simulink model "c00017M_harness"  (R2018a)
settings: Solver=FixedStepAuto  StartTime=0.0  StopTime=300  FixedStep=0.1  RelTol=1e-3
undefined symbols (not defined in the file): A1, hmax, R1, R2, sigbuilder_block
(part 1 of 6)
settings Model: Creator=aarrieta  LastModifiedBy=umarkiegi

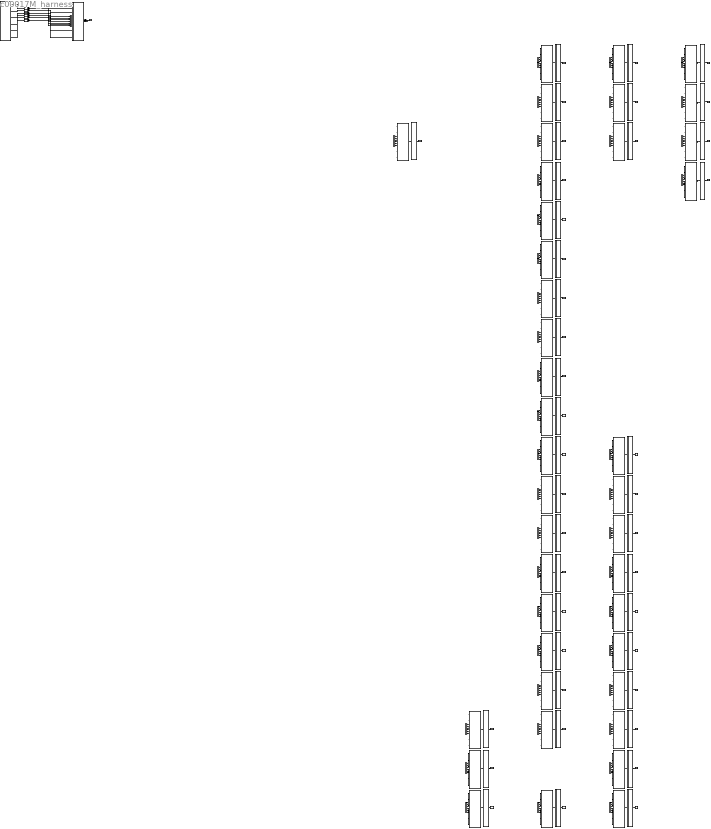
== system c00017M_harness ==
  CPSUT : Subsystem
  Eval117 : Subsystem
  Eval118 : Subsystem
  Eval119 : Subsystem
  Eval120 : Subsystem
  Eval121 : Subsystem
  Eval122 : Subsystem
  Eval123 : Subsystem
  Eval124 : Subsystem
  Eval125 : Subsystem
  Eval126 : Subsystem
  Eval127 : Subsystem
  Eval128 : Subsystem
  Eval129 : Subsystem
  Eval130 : Subsystem
  Eval131 : Subsystem
  Eval132 : Subsystem
  Eval133 : Subsystem
  Eval134 : Subsystem
  Eval135 : Subsystem
  Eval136 : Subsystem
  Eval137 : Subsystem
  Eval139 : Subsystem
  Eval140 : Subsystem
  Eval141 : Subsystem
  Eval142 : Subsystem
  Eval150 : Subsystem
  Eval151 : Subsystem
  Eval152 : Subsystem
  Eval153 : Subsystem
  Eval154 : Subsystem
  Eval155 : Subsystem
  Eval156 : Subsystem
  Eval157 : Subsystem
  Eval158 : Subsystem
  Eval159 : Subsystem
  Eval160 : Subsystem
  Eval161 : Subsystem
  Eval162 : Subsystem
  Eval163 : Subsystem
  Eval82 : Subsystem
  Inputs : Subsystem  Tag=STV Subsys  LoadFcn=sigbuilder_block('load');  StartFcn=sigbuilder_block('start');  StopFcn=sigbuilder_block('stop');  ClipboardFcn=sigbuilder_block('clipboard');  mask(Sigbuilder block){tuvar=[0:10]}
      mask init:
      | if ~strcmp(get_param(bdroot(gcb),'SimulationStatus'),'stopped'),tuvar = sigbuilder_block('maskInit'); end
      settings: CopyFcn=sigbuilder_block('copy');  DeleteFcn=sigbuilder_block('delete');  ModelCloseFcn=sigbuilder_block('modelClose');  PreSaveFcn=sigbuilder_block('preSave');  PauseFcn=sigbuilder_block('pause');  ContinueFcn=sigbuilder_block('continue');  NameChangeFcn=sigbuilder_block('namechange');  OpenFcn=sigbuilder_block('open',[276.75 163.5 675.75 486.75 ]);  CloseFcn=sigbuilder_block('close');
      mask Display: plot(0, 0, 100, 100,[2, 2, 32, 32, 2], [68, 8, 8, 68, 68],[32, 2], [38, 38], [32, 19, 2],[53, 60, 44], [32, 17, 17, 2],[16, 16, 31, 31]);txt = getActiveGroup(gcbh);text(2, 100, txt,'verticalAlignment', 'top');
  M083 : Subsystem
  M118 : Subsystem
  M119 : Subsystem
  M120 : Subsystem
  M121 : Subsystem
  M122 : Subsystem
  M123 : Subsystem
  M124 : Subsystem
  M125 : Subsystem
  M126 : Subsystem
  M127 : Subsystem
  M128 : Subsystem
  M129 : Subsystem
  M130 : Subsystem
  M131 : Subsystem
  M132 : Subsystem
  M133 : Subsystem
  M134 : Subsystem
  M135 : Subsystem
  M136 : Subsystem
  M137 : Subsystem
  M138 : Subsystem
  M140 : Subsystem
  M141 : Subsystem
  M142 : Subsystem
  M143 : Subsystem
  M151 : Subsystem
  M152 : Subsystem
  M153 : Subsystem
  M154 : Subsystem
  M155 : Subsystem
  M156 : Subsystem
  M157 : Subsystem
  M158 : Subsystem
  M159 : Subsystem
  M160 : Subsystem
  M161 : Subsystem
  M162 : Subsystem
  M163 : Subsystem
  M164 : Subsystem
  To Workspace117 : ToWorkspace  VariableName=mutant118  SampleTime=-1
  To Workspace118 : ToWorkspace  VariableName=mutant119  SampleTime=-1
  To Workspace119 : ToWorkspace  VariableName=mutant120  SampleTime=-1
  To Workspace120 : ToWorkspace  VariableName=mutant121  SampleTime=-1
  To Workspace121 : ToWorkspace  VariableName=mutant122  SampleTime=-1
  To Workspace122 : ToWorkspace  VariableName=mutant123  SampleTime=-1
  To Workspace123 : ToWorkspace  VariableName=mutant124  SampleTime=-1
  To Workspace124 : ToWorkspace  VariableName=mutant125  SampleTime=-1
  To Workspace125 : ToWorkspace  VariableName=mutant126  SampleTime=-1
  To Workspace126 : ToWorkspace  VariableName=mutant127  SampleTime=-1
  To Workspace127 : ToWorkspace  VariableName=mutant128  SampleTime=-1
  To Workspace128 : ToWorkspace  VariableName=mutant129  SampleTime=-1
  To Workspace129 : ToWorkspace  VariableName=mutant130  SampleTime=-1
  To Workspace130 : ToWorkspace  VariableName=mutant131  SampleTime=-1
  To Workspace131 : ToWorkspace  VariableName=mutant132  SampleTime=-1
  To Workspace132 : ToWorkspace  VariableName=mutant133  SampleTime=-1
  To Workspace133 : ToWorkspace  VariableName=mutant134  SampleTime=-1
  To Workspace134 : ToWorkspace  VariableName=mutant135  SampleTime=-1
  To Workspace135 : ToWorkspace  VariableName=mutant136  SampleTime=-1
  To Workspace136 : ToWorkspace  VariableName=mutant137  SampleTime=-1
  To Workspace137 : ToWorkspace  VariableName=mutant138  SampleTime=-1
  To Workspace139 : ToWorkspace  VariableName=mutant140  SampleTime=-1
  To Workspace140 : ToWorkspace  VariableName=mutant141  SampleTime=-1
  To Workspace141 : ToWorkspace  VariableName=mutant142  SampleTime=-1
  To Workspace142 : ToWorkspace  VariableName=mutant143  SampleTime=-1
  To Workspace150 : ToWorkspace  VariableName=mutant151  SampleTime=-1
  To Workspace151 : ToWorkspace  VariableName=mutant152  SampleTime=-1
  To Workspace152 : ToWorkspace  VariableName=mutant153  SampleTime=-1
  To Workspace153 : ToWorkspace  VariableName=mutant154  SampleTime=-1
  To Workspace154 : ToWorkspace  VariableName=mutant155  SampleTime=-1
  To Workspace155 : ToWorkspace  VariableName=mutant156  SampleTime=-1
  To Workspace156 : ToWorkspace  VariableName=mutant157  SampleTime=-1
  To Workspace157 : ToWorkspace  VariableName=mutant158  SampleTime=-1
  To Workspace158 : ToWorkspace  VariableName=mutant159  SampleTime=-1
  To Workspace159 : ToWorkspace  VariableName=mutant160  SampleTime=-1
  To Workspace160 : ToWorkspace  VariableName=mutant161  SampleTime=-1
  To Workspace161 : ToWorkspace  VariableName=mutant162  SampleTime=-1
  To Workspace162 : ToWorkspace  VariableName=mutant163  SampleTime=-1
  To Workspace163 : ToWorkspace  VariableName=mutant164  SampleTime=-1
  To Workspace82 : ToWorkspace  VariableName=mutant083  SampleTime=-1
  dtc_CT2 : DataTypeConversion
  dtc_E2 : DataTypeConversion
  dtc_EB2 : DataTypeConversion
  dtc_F2 : DataTypeConversion
  dtc_MR2 : DataTypeConversion
  dtc_T2 : DataTypeConversion
  LL2 : Outport
  tag scope: out2=global
  wires:
  CPSUT/1(LL2) -> [out2], LL2/1
  [in7] -> M083/1(CT2)
  [in8] -> M083/2(F2)
  [in9] -> M083/3(E2)
  [in10] -> M083/4(MR2)
  [in11] -> M083/5(T2)
  [in12] -> M083/6(EB2)
  M083/1(LL2) -> Eval82/1(In2)
  Eval82/1(Out1) -> To Workspace82/1
  [in7] -> M118/1(CT2)
  [in8] -> M118/2(F2)
  [in9] -> M118/3(E2)
  [in10] -> M118/4(MR2)
  [in11] -> M118/5(T2)
  [in12] -> M118/6(EB2)
  M118/1(LL2) -> Eval117/1(In2)
  Eval117/1(Out1) -> To Workspace117/1
  [in7] -> M119/1(CT2)
  [in8] -> M119/2(F2)
  [in9] -> M119/3(E2)
  [in10] -> M119/4(MR2)
  [in11] -> M119/5(T2)
  [in12] -> M119/6(EB2)
  M119/1(LL2) -> Eval118/1(In2)
  Eval118/1(Out1) -> To Workspace118/1
  [in7] -> M120/1(CT2)
  [in8] -> M120/2(F2)
  [in9] -> M120/3(E2)
  [in10] -> M120/4(MR2)
  [in11] -> M120/5(T2)
  [in12] -> M120/6(EB2)
  M120/1(LL2) -> Eval119/1(In2)
  Eval119/1(Out1) -> To Workspace119/1
  [in7] -> M121/1(CT2)
  [in8] -> M121/2(F2)
  [in9] -> M121/3(E2)
  [in10] -> M121/4(MR2)
  [in11] -> M121/5(T2)
  [in12] -> M121/6(EB2)
  M121/1(LL2) -> Eval120/1(In2)
  Eval120/1(Out1) -> To Workspace120/1
  [in7] -> M122/1(CT2)
  [in8] -> M122/2(F2)
  [in9] -> M122/3(E2)
  [in10] -> M122/4(MR2)
  [in11] -> M122/5(T2)
  [in12] -> M122/6(EB2)
  M122/1(LL2) -> Eval121/1(In2)
  Eval121/1(Out1) -> To Workspace121/1
  [in7] -> M123/1(CT2)
  [in8] -> M123/2(F2)
  [in9] -> M123/3(E2)
  [in10] -> M123/4(MR2)
  [in11] -> M123/5(T2)
  [in12] -> M123/6(EB2)
  M123/1(LL2) -> Eval122/1(In2)
  Eval122/1(Out1) -> To Workspace122/1
  [in7] -> M124/1(CT2)
  [in8] -> M124/2(F2)
  [in9] -> M124/3(E2)
  [in10] -> M124/4(MR2)
  [in11] -> M124/5(T2)
  [in12] -> M124/6(EB2)
  M124/1(LL2) -> Eval123/1(In2)
  Eval123/1(Out1) -> To Workspace123/1
  [in7] -> M125/1(CT2)
  [in8] -> M125/2(F2)
  [in9] -> M125/3(E2)
  [in10] -> M125/4(MR2)
  [in11] -> M125/5(T2)
  [in12] -> M125/6(EB2)
  M125/1(LL2) -> Eval124/1(In2)
  Eval124/1(Out1) -> To Workspace124/1
  [in7] -> M126/1(CT2)
  [in8] -> M126/2(F2)
  [in9] -> M126/3(E2)
  [in10] -> M126/4(MR2)
  [in11] -> M126/5(T2)
  [in12] -> M126/6(EB2)
  M126/1(LL2) -> Eval125/1(In2)
  Eval125/1(Out1) -> To Workspace125/1
  [in7] -> M127/1(CT2)
  [in8] -> M127/2(F2)
  [in9] -> M127/3(E2)
  [in10] -> M127/4(MR2)
  [in11] -> M127/5(T2)
  [in12] -> M127/6(EB2)
  M127/1(LL2) -> Eval126/1(In2)
  Eval126/1(Out1) -> To Workspace126/1
  [in7] -> M128/1(CT2)
  [in8] -> M128/2(F2)
  [in9] -> M128/3(E2)
  [in10] -> M128/4(MR2)
  [in11] -> M128/5(T2)
  [in12] -> M128/6(EB2)
  M128/1(LL2) -> Eval127/1(In2)
  Eval127/1(Out1) -> To Workspace127/1
  [in7] -> M129/1(CT2)
  [in8] -> M129/2(F2)
  [in9] -> M129/3(E2)
  [in10] -> M129/4(MR2)
  [in11] -> M129/5(T2)
  [in12] -> M129/6(EB2)
  M129/1(LL2) -> Eval128/1(In2)
  Eval128/1(Out1) -> To Workspace128/1
  [in7] -> M130/1(CT2)
  [in8] -> M130/2(F2)
  [in9] -> M130/3(E2)
  [in10] -> M130/4(MR2)
  [in11] -> M130/5(T2)
  [in12] -> M130/6(EB2)
  M130/1(LL2) -> Eval129/1(In2)
  Eval129/1(Out1) -> To Workspace129/1
  [in7] -> M131/1(CT2)
  [in8] -> M131/2(F2)
  [in9] -> M131/3(E2)
  [in10] -> M131/4(MR2)
  [in11] -> M131/5(T2)
  [in12] -> M131/6(EB2)
  M131/1(LL2) -> Eval130/1(In2)
  Eval130/1(Out1) -> To Workspace130/1
  [in7] -> M132/1(CT2)
  [in8] -> M132/2(F2)
  [in9] -> M132/3(E2)
  [in10] -> M132/4(MR2)
  [in11] -> M132/5(T2)
  [in12] -> M132/6(EB2)
  M132/1(LL2) -> Eval131/1(In2)
  Eval131/1(Out1) -> To Workspace131/1
  [in7] -> M133/1(CT2)
  [in8] -> M133/2(F2)
  [in9] -> M133/3(E2)
  [in10] -> M133/4(MR2)
  [in11] -> M133/5(T2)
  [in12] -> M133/6(EB2)
  M133/1(LL2) -> Eval132/1(In2)
  Eval132/1(Out1) -> To Workspace132/1
  [in7] -> M134/1(CT2)
  [in8] -> M134/2(F2)
  [in9] -> M134/3(E2)
  [in10] -> M134/4(MR2)
  [in11] -> M134/5(T2)
  [in12] -> M134/6(EB2)
  M134/1(LL2) -> Eval133/1(In2)
  Eval133/1(Out1) -> To Workspace133/1
  [in7] -> M135/1(CT2)
  [in8] -> M135/2(F2)
  [in9] -> M135/3(E2)
  [in10] -> M135/4(MR2)
  [in11] -> M135/5(T2)
  [in12] -> M135/6(EB2)
  M135/1(LL2) -> Eval134/1(In2)
  Eval134/1(Out1) -> To Workspace134/1
  [in7] -> M136/1(CT2)
  [in8] -> M136/2(F2)
  [in9] -> M136/3(E2)
  [in10] -> M136/4(MR2)
  [in11] -> M136/5(T2)
  [in12] -> M136/6(EB2)
  M136/1(LL2) -> Eval135/1(In2)
  Eval135/1(Out1) -> To Workspace135/1
  [in7] -> M137/1(CT2)
  [in8] -> M137/2(F2)
  [in9] -> M137/3(E2)
  [in10] -> M137/4(MR2)
  [in11] -> M137/5(T2)
  [in12] -> M137/6(EB2)
  M137/1(LL2) -> Eval136/1(In2)
  Eval136/1(Out1) -> To Workspace136/1
  [in7] -> M138/1(CT2)
  [in8] -> M138/2(F2)
  [in9] -> M138/3(E2)
  [in10] -> M138/4(MR2)
  [in11] -> M138/5(T2)
  [in12] -> M138/6(EB2)
  M138/1(LL2) -> Eval137/1(In2)
  Eval137/1(Out1) -> To Workspace137/1
  [in7] -> M140/1(CT2)
  [in8] -> M140/2(F2)
  [in9] -> M140/3(E2)
  [in10] -> M140/4(MR2)
  [in11] -> M140/5(T2)
  [in12] -> M140/6(EB2)
  M140/1(LL2) -> Eval139/1(In2)
  Eval139/1(Out1) -> To Workspace139/1
  [in7] -> M141/1(CT2)
  [in8] -> M141/2(F2)
  [in9] -> M141/3(E2)
  [in10] -> M141/4(MR2)
  [in11] -> M141/5(T2)
  [in12] -> M141/6(EB2)
  M141/1(LL2) -> Eval140/1(In2)
  Eval140/1(Out1) -> To Workspace140/1
  [in7] -> M142/1(CT2)
  [in8] -> M142/2(F2)
  [in9] -> M142/3(E2)
  [in10] -> M142/4(MR2)
  [in11] -> M142/5(T2)
  [in12] -> M142/6(EB2)
  M142/1(LL2) -> Eval141/1(In2)
  Eval141/1(Out1) -> To Workspace141/1
  [in7] -> M143/1(CT2)
  [in8] -> M143/2(F2)
  [in9] -> M143/3(E2)
  [in10] -> M143/4(MR2)
  [in11] -> M143/5(T2)
  [in12] -> M143/6(EB2)
  M143/1(LL2) -> Eval142/1(In2)
  Eval142/1(Out1) -> To Workspace142/1
  [in7] -> M151/1(CT2)
  [in8] -> M151/2(F2)
  [in9] -> M151/3(E2)
  [in10] -> M151/4(MR2)
  [in11] -> M151/5(T2)
  [in12] -> M151/6(EB2)
  M151/1(LL2) -> Eval150/1(In2)
  Eval150/1(Out1) -> To Workspace150/1
  [in7] -> M152/1(CT2)
  [in8] -> M152/2(F2)
  [in9] -> M152/3(E2)
  [in10] -> M152/4(MR2)
  [in11] -> M152/5(T2)
  [in12] -> M152/6(EB2)
  M152/1(LL2) -> Eval151/1(In2)
  Eval151/1(Out1) -> To Workspace151/1
  [in7] -> M153/1(CT2)
  [in8] -> M153/2(F2)
  [in9] -> M153/3(E2)
  [in10] -> M153/4(MR2)
  [in11] -> M153/5(T2)
  [in12] -> M153/6(EB2)
  M153/1(LL2) -> Eval152/1(In2)
  Eval152/1(Out1) -> To Workspace152/1
  [in7] -> M154/1(CT2)
  [in8] -> M154/2(F2)
  [in9] -> M154/3(E2)
  [in10] -> M154/4(MR2)
  [in11] -> M154/5(T2)
  [in12] -> M154/6(EB2)
  M154/1(LL2) -> Eval153/1(In2)
  Eval153/1(Out1) -> To Workspace153/1
  [in7] -> M155/1(CT2)
  [in8] -> M155/2(F2)
  [in9] -> M155/3(E2)
  [in10] -> M155/4(MR2)
  [in11] -> M155/5(T2)
  [in12] -> M155/6(EB2)
  M155/1(LL2) -> Eval154/1(In2)
  Eval154/1(Out1) -> To Workspace154/1
  [in7] -> M156/1(CT2)
  [in8] -> M156/2(F2)
  [in9] -> M156/3(E2)
  [in10] -> M156/4(MR2)
  [in11] -> M156/5(T2)
  [in12] -> M156/6(EB2)
  M156/1(LL2) -> Eval155/1(In2)
  Eval155/1(Out1) -> To Workspace155/1
  [in7] -> M157/1(CT2)
  [in8] -> M157/2(F2)
  [in9] -> M157/3(E2)
  [in10] -> M157/4(MR2)
  [in11] -> M157/5(T2)
  [in12] -> M157/6(EB2)
  M157/1(LL2) -> Eval156/1(In2)
  Eval156/1(Out1) -> To Workspace156/1
  [in7] -> M158/1(CT2)
  [in8] -> M158/2(F2)
  [in9] -> M158/3(E2)
  [in10] -> M158/4(MR2)
  [in11] -> M158/5(T2)
  [in12] -> M158/6(EB2)
  M158/1(LL2) -> Eval157/1(In2)
  Eval157/1(Out1) -> To Workspace157/1
  [in7] -> M159/1(CT2)
  [in8] -> M159/2(F2)
  [in9] -> M159/3(E2)
  [in10] -> M159/4(MR2)
  [in11] -> M159/5(T2)
  [in12] -> M159/6(EB2)
  M159/1(LL2) -> Eval158/1(In2)
  Eval158/1(Out1) -> To Workspace158/1
  [in7] -> M160/1(CT2)
  [in8] -> M160/2(F2)
  [in9] -> M160/3(E2)
  [in10] -> M160/4(MR2)
  [in11] -> M160/5(T2)
  [in12] -> M160/6(EB2)
  M160/1(LL2) -> Eval159/1(In2)
  Eval159/1(Out1) -> To Workspace159/1
  [in7] -> M161/1(CT2)
  [in8] -> M161/2(F2)
  [in9] -> M161/3(E2)
  [in10] -> M161/4(MR2)
  [in11] -> M161/5(T2)
  [in12] -> M161/6(EB2)
  M161/1(LL2) -> Eval160/1(In2)
  Eval160/1(Out1) -> To Workspace160/1
  [in7] -> M162/1(CT2)
  [in8] -> M162/2(F2)
  [in9] -> M162/3(E2)
  [in10] -> M162/4(MR2)
  [in11] -> M162/5(T2)
  [in12] -> M162/6(EB2)
  M162/1(LL2) -> Eval161/1(In2)
  Eval161/1(Out1) -> To Workspace161/1
  [in7] -> M163/1(CT2)
  [in8] -> M163/2(F2)
  [in9] -> M163/3(E2)
  [in10] -> M163/4(MR2)
  [in11] -> M163/5(T2)
  [in12] -> M163/6(EB2)
  M163/1(LL2) -> Eval162/1(In2)
  Eval162/1(Out1) -> To Workspace162/1
  [in7] -> M164/1(CT2)
  [in8] -> M164/2(F2)
  [in9] -> M164/3(E2)
  [in10] -> M164/4(MR2)
  [in11] -> M164/5(T2)
  [in12] -> M164/6(EB2)
  M164/1(LL2) -> Eval163/1(In2)
  Eval163/1(Out1) -> To Workspace163/1
  Inputs/1(CT2) -> dtc_CT2/1
  dtc_CT2/1 -> CPSUT/1(CT2), [in7]
  Inputs/2(F2) -> dtc_F2/1
  dtc_F2/1 -> CPSUT/2(F2), [in8]
  Inputs/3(E2) -> dtc_E2/1
  dtc_E2/1 -> CPSUT/3(E2), [in9]
  Inputs/4(MR2) -> dtc_MR2/1
  dtc_MR2/1 -> CPSUT/4(MR2), [in10]
  Inputs/5(T2) -> dtc_T2/1
  dtc_T2/1 -> CPSUT/5(T2), [in11]
  Inputs/6(EB2) -> dtc_EB2/1
  dtc_EB2/1 -> CPSUT/6(EB2), [in12]

== system c00017M_harness/CPSUT ==
  note: VALUES
      | ---------------------------------
      | ControlType = 1 | 2 | 3
      | FillTank = 0 | 1
      | EmptyTank = 0 | 1
      | ManualReference between 0 and 1
      | Tempreature between 0 and 100
      | EmergencyButton = 0 | 1
      | LiquidLevel between 0 and 1 (hmax)
  note: Inputs For Tank2
  note: NAMES
      | --------------------------------------------
      | CT1 = ControlType Tank 1
      | F1 = Fill Tank 1
      | E1 = Empty Tank 1
      | MR1 = Manual Reference Tank1
      | T1 = Temperature Tank 1
      | EB1 = Emergency Button Tank 1
      | LL1 = Liquid Level 1
  note: Inputs For Tank3
  note: Inputs For Tank1
  CT2 : Inport
  F2 : Inport  Port=2
  E2 : Inport  Port=3
  MR2 : Inport  Port=4
  T2 : Inport  Port=5
  EB2 : Inport  Port=6
  Tank2 : Subsystem
  LL2 : Outport
  wires:
  Tank2/1(LL2) -> LL2/1
  EB2/1 -> Tank2/6(EB2)
  CT2/1 -> Tank2/1(CT2)
  F2/1 -> Tank2/2(F2)
  E2/1 -> Tank2/3(E2)
  T2/1 -> Tank2/5(T2)
  MR2/1 -> Tank2/4(MR2)

== system c00017M_harness/Eval117 ==
  In2 : Inport
  Constant1 : Constant
  Constant3 : Constant
  Data Type Conversion1 : DataTypeConversion
  Memory2 : Memory  InitialCondition=1
  MinMax : MinMax  Inputs=3
  MinMax2 : MinMax  Inputs=2
  ROOut2 : RelationalOperator  Operator===  OutDataTypeStr=boolean  RndMeth=Simplest
  Out1 : Outport
  wires:
  Data Type Conversion1/1 -> MinMax2/1
  MinMax2/1 -> MinMax/2, Memory2/1
  Memory2/1 -> MinMax2/2
  ROOut2/1 -> Data Type Conversion1/1
  [out2] -> ROOut2/2
  In2/1 -> ROOut2/1
  MinMax/1 -> Out1/1
  Constant1/1 -> MinMax/1
  Constant3/1 -> MinMax/3

== system c00017M_harness/Eval118 ==
  In2 : Inport
  Constant1 : Constant
  Constant3 : Constant
  Data Type Conversion1 : DataTypeConversion
  Memory2 : Memory  InitialCondition=1
  MinMax : MinMax  Inputs=3
  MinMax2 : MinMax  Inputs=2
  ROOut2 : RelationalOperator  Operator===  OutDataTypeStr=boolean  RndMeth=Simplest
  Out1 : Outport
  wires:
  Data Type Conversion1/1 -> MinMax2/1
  MinMax2/1 -> MinMax/2, Memory2/1
  Memory2/1 -> MinMax2/2
  ROOut2/1 -> Data Type Conversion1/1
  [out2] -> ROOut2/2
  In2/1 -> ROOut2/1
  MinMax/1 -> Out1/1
  Constant1/1 -> MinMax/1
  Constant3/1 -> MinMax/3

== system c00017M_harness/Eval119 ==
  In2 : Inport
  Constant1 : Constant
  Constant3 : Constant
  Data Type Conversion1 : DataTypeConversion
  Memory2 : Memory  InitialCondition=1
  MinMax : MinMax  Inputs=3
  MinMax2 : MinMax  Inputs=2
  ROOut2 : RelationalOperator  Operator===  OutDataTypeStr=boolean  RndMeth=Simplest
  Out1 : Outport
  wires:
  Data Type Conversion1/1 -> MinMax2/1
  MinMax2/1 -> MinMax/2, Memory2/1
  Memory2/1 -> MinMax2/2
  ROOut2/1 -> Data Type Conversion1/1
  [out2] -> ROOut2/2
  In2/1 -> ROOut2/1
  MinMax/1 -> Out1/1
  Constant1/1 -> MinMax/1
  Constant3/1 -> MinMax/3

== system c00017M_harness/Eval120 ==
  In2 : Inport
  Constant1 : Constant
  Constant3 : Constant
  Data Type Conversion1 : DataTypeConversion
  Memory2 : Memory  InitialCondition=1
  MinMax : MinMax  Inputs=3
  MinMax2 : MinMax  Inputs=2
  ROOut2 : RelationalOperator  Operator===  OutDataTypeStr=boolean  RndMeth=Simplest
  Out1 : Outport
  wires:
  Data Type Conversion1/1 -> MinMax2/1
  MinMax2/1 -> MinMax/2, Memory2/1
  Memory2/1 -> MinMax2/2
  ROOut2/1 -> Data Type Conversion1/1
  [out2] -> ROOut2/2
  In2/1 -> ROOut2/1
  MinMax/1 -> Out1/1
  Constant1/1 -> MinMax/1
  Constant3/1 -> MinMax/3

== system c00017M_harness/Eval121 ==
  In2 : Inport
  Constant1 : Constant
  Constant3 : Constant
  Data Type Conversion1 : DataTypeConversion
  Memory2 : Memory  InitialCondition=1
  MinMax : MinMax  Inputs=3
  MinMax2 : MinMax  Inputs=2
  ROOut2 : RelationalOperator  Operator===  OutDataTypeStr=boolean  RndMeth=Simplest
  Out1 : Outport
  wires:
  Data Type Conversion1/1 -> MinMax2/1
  MinMax2/1 -> MinMax/2, Memory2/1
  Memory2/1 -> MinMax2/2
  ROOut2/1 -> Data Type Conversion1/1
  [out2] -> ROOut2/2
  In2/1 -> ROOut2/1
  MinMax/1 -> Out1/1
  Constant1/1 -> MinMax/1
  Constant3/1 -> MinMax/3

== system c00017M_harness/Eval122 ==
  In2 : Inport
  Constant1 : Constant
  Constant3 : Constant
  Data Type Conversion1 : DataTypeConversion
  Memory2 : Memory  InitialCondition=1
  MinMax : MinMax  Inputs=3
  MinMax2 : MinMax  Inputs=2
  ROOut2 : RelationalOperator  Operator===  OutDataTypeStr=boolean  RndMeth=Simplest
  Out1 : Outport
  wires:
  Data Type Conversion1/1 -> MinMax2/1
  MinMax2/1 -> MinMax/2, Memory2/1
  Memory2/1 -> MinMax2/2
  ROOut2/1 -> Data Type Conversion1/1
  [out2] -> ROOut2/2
  In2/1 -> ROOut2/1
  MinMax/1 -> Out1/1
  Constant1/1 -> MinMax/1
  Constant3/1 -> MinMax/3

== system c00017M_harness/Eval123 ==
  In2 : Inport
  Constant1 : Constant
  Constant3 : Constant
  Data Type Conversion1 : DataTypeConversion
  Memory2 : Memory  InitialCondition=1
  MinMax : MinMax  Inputs=3
  MinMax2 : MinMax  Inputs=2
  ROOut2 : RelationalOperator  Operator===  OutDataTypeStr=boolean  RndMeth=Simplest
  Out1 : Outport
  wires:
  Data Type Conversion1/1 -> MinMax2/1
  MinMax2/1 -> MinMax/2, Memory2/1
  Memory2/1 -> MinMax2/2
  ROOut2/1 -> Data Type Conversion1/1
  [out2] -> ROOut2/2
  In2/1 -> ROOut2/1
  MinMax/1 -> Out1/1
  Constant1/1 -> MinMax/1
  Constant3/1 -> MinMax/3

== system c00017M_harness/Eval124 ==
  In2 : Inport
  Constant1 : Constant
  Constant3 : Constant
  Data Type Conversion1 : DataTypeConversion
  Memory2 : Memory  InitialCondition=1
  MinMax : MinMax  Inputs=3
  MinMax2 : MinMax  Inputs=2
  ROOut2 : RelationalOperator  Operator===  OutDataTypeStr=boolean  RndMeth=Simplest
  Out1 : Outport
  wires:
  Data Type Conversion1/1 -> MinMax2/1
  MinMax2/1 -> MinMax/2, Memory2/1
  Memory2/1 -> MinMax2/2
  ROOut2/1 -> Data Type Conversion1/1
  [out2] -> ROOut2/2
  In2/1 -> ROOut2/1
  MinMax/1 -> Out1/1
  Constant1/1 -> MinMax/1
  Constant3/1 -> MinMax/3

== system c00017M_harness/Eval125 ==
  In2 : Inport
  Constant1 : Constant
  Constant3 : Constant
  Data Type Conversion1 : DataTypeConversion
  Memory2 : Memory  InitialCondition=1
  MinMax : MinMax  Inputs=3
  MinMax2 : MinMax  Inputs=2
  ROOut2 : RelationalOperator  Operator===  OutDataTypeStr=boolean  RndMeth=Simplest
  Out1 : Outport
  wires:
  Data Type Conversion1/1 -> MinMax2/1
  MinMax2/1 -> MinMax/2, Memory2/1
  Memory2/1 -> MinMax2/2
  ROOut2/1 -> Data Type Conversion1/1
  [out2] -> ROOut2/2
  In2/1 -> ROOut2/1
  MinMax/1 -> Out1/1
  Constant1/1 -> MinMax/1
  Constant3/1 -> MinMax/3

== system c00017M_harness/Eval126 ==
  In2 : Inport
  Constant1 : Constant
  Constant3 : Constant
  Data Type Conversion1 : DataTypeConversion
  Memory2 : Memory  InitialCondition=1
  MinMax : MinMax  Inputs=3
  MinMax2 : MinMax  Inputs=2
  ROOut2 : RelationalOperator  Operator===  OutDataTypeStr=boolean  RndMeth=Simplest
  Out1 : Outport
  wires:
  Data Type Conversion1/1 -> MinMax2/1
  MinMax2/1 -> MinMax/2, Memory2/1
  Memory2/1 -> MinMax2/2
  ROOut2/1 -> Data Type Conversion1/1
  [out2] -> ROOut2/2
  In2/1 -> ROOut2/1
  MinMax/1 -> Out1/1
  Constant1/1 -> MinMax/1
  Constant3/1 -> MinMax/3

== system c00017M_harness/Eval127 ==
  In2 : Inport
  Constant1 : Constant
  Constant3 : Constant
  Data Type Conversion1 : DataTypeConversion
  Memory2 : Memory  InitialCondition=1
  MinMax : MinMax  Inputs=3
  MinMax2 : MinMax  Inputs=2
  ROOut2 : RelationalOperator  Operator===  OutDataTypeStr=boolean  RndMeth=Simplest
  Out1 : Outport
  wires:
  Data Type Conversion1/1 -> MinMax2/1
  MinMax2/1 -> MinMax/2, Memory2/1
  Memory2/1 -> MinMax2/2
  ROOut2/1 -> Data Type Conversion1/1
  [out2] -> ROOut2/2
  In2/1 -> ROOut2/1
  MinMax/1 -> Out1/1
  Constant1/1 -> MinMax/1
  Constant3/1 -> MinMax/3

== system c00017M_harness/Eval128 ==
  In2 : Inport
  Constant1 : Constant
  Constant3 : Constant
  Data Type Conversion1 : DataTypeConversion
  Memory2 : Memory  InitialCondition=1
  MinMax : MinMax  Inputs=3
  MinMax2 : MinMax  Inputs=2
  ROOut2 : RelationalOperator  Operator===  OutDataTypeStr=boolean  RndMeth=Simplest
  Out1 : Outport
  wires:
  Data Type Conversion1/1 -> MinMax2/1
  MinMax2/1 -> MinMax/2, Memory2/1
  Memory2/1 -> MinMax2/2
  ROOut2/1 -> Data Type Conversion1/1
  [out2] -> ROOut2/2
  In2/1 -> ROOut2/1
  MinMax/1 -> Out1/1
  Constant1/1 -> MinMax/1
  Constant3/1 -> MinMax/3

== system c00017M_harness/Eval129 ==
  In2 : Inport
  Constant1 : Constant
  Constant3 : Constant
  Data Type Conversion1 : DataTypeConversion
  Memory2 : Memory  InitialCondition=1
  MinMax : MinMax  Inputs=3
  MinMax2 : MinMax  Inputs=2
  ROOut2 : RelationalOperator  Operator===  OutDataTypeStr=boolean  RndMeth=Simplest
  Out1 : Outport
  wires:
  Data Type Conversion1/1 -> MinMax2/1
  MinMax2/1 -> MinMax/2, Memory2/1
  Memory2/1 -> MinMax2/2
  ROOut2/1 -> Data Type Conversion1/1
  [out2] -> ROOut2/2
  In2/1 -> ROOut2/1
  MinMax/1 -> Out1/1
  Constant1/1 -> MinMax/1
  Constant3/1 -> MinMax/3

== system c00017M_harness/Eval130 ==
  In2 : Inport
  Constant1 : Constant
  Constant3 : Constant
  Data Type Conversion1 : DataTypeConversion
  Memory2 : Memory  InitialCondition=1
  MinMax : MinMax  Inputs=3
  MinMax2 : MinMax  Inputs=2
  ROOut2 : RelationalOperator  Operator===  OutDataTypeStr=boolean  RndMeth=Simplest
  Out1 : Outport
  wires:
  Data Type Conversion1/1 -> MinMax2/1
  MinMax2/1 -> MinMax/2, Memory2/1
  Memory2/1 -> MinMax2/2
  ROOut2/1 -> Data Type Conversion1/1
  [out2] -> ROOut2/2
  In2/1 -> ROOut2/1
  MinMax/1 -> Out1/1
  Constant1/1 -> MinMax/1
  Constant3/1 -> MinMax/3

== system c00017M_harness/Eval131 ==
  In2 : Inport
  Constant1 : Constant
  Constant3 : Constant
  Data Type Conversion1 : DataTypeConversion
  Memory2 : Memory  InitialCondition=1
  MinMax : MinMax  Inputs=3
  MinMax2 : MinMax  Inputs=2
  ROOut2 : RelationalOperator  Operator===  OutDataTypeStr=boolean  RndMeth=Simplest
  Out1 : Outport
  wires:
  Data Type Conversion1/1 -> MinMax2/1
  MinMax2/1 -> MinMax/2, Memory2/1
  Memory2/1 -> MinMax2/2
  ROOut2/1 -> Data Type Conversion1/1
  [out2] -> ROOut2/2
  In2/1 -> ROOut2/1
  MinMax/1 -> Out1/1
  Constant1/1 -> MinMax/1
  Constant3/1 -> MinMax/3

== system c00017M_harness/Eval132 ==
  In2 : Inport
  Constant1 : Constant
  Constant3 : Constant
  Data Type Conversion1 : DataTypeConversion
  Memory2 : Memory  InitialCondition=1
  MinMax : MinMax  Inputs=3
  MinMax2 : MinMax  Inputs=2
  ROOut2 : RelationalOperator  Operator===  OutDataTypeStr=boolean  RndMeth=Simplest
  Out1 : Outport
  wires:
  Data Type Conversion1/1 -> MinMax2/1
  MinMax2/1 -> MinMax/2, Memory2/1
  Memory2/1 -> MinMax2/2
  ROOut2/1 -> Data Type Conversion1/1
  [out2] -> ROOut2/2
  In2/1 -> ROOut2/1
  MinMax/1 -> Out1/1
  Constant1/1 -> MinMax/1
  Constant3/1 -> MinMax/3

== system c00017M_harness/Eval133 ==
  In2 : Inport
  Constant1 : Constant
  Constant3 : Constant
  Data Type Conversion1 : DataTypeConversion
  Memory2 : Memory  InitialCondition=1
  MinMax : MinMax  Inputs=3
  MinMax2 : MinMax  Inputs=2
  ROOut2 : RelationalOperator  Operator===  OutDataTypeStr=boolean  RndMeth=Simplest
  Out1 : Outport
  wires:
  Data Type Conversion1/1 -> MinMax2/1
  MinMax2/1 -> MinMax/2, Memory2/1
  Memory2/1 -> MinMax2/2
  ROOut2/1 -> Data Type Conversion1/1
  [out2] -> ROOut2/2
  In2/1 -> ROOut2/1
  MinMax/1 -> Out1/1
  Constant1/1 -> MinMax/1
  Constant3/1 -> MinMax/3

== system c00017M_harness/Eval134 ==
  In2 : Inport
  Constant1 : Constant
  Constant3 : Constant
  Data Type Conversion1 : DataTypeConversion
  Memory2 : Memory  InitialCondition=1
  MinMax : MinMax  Inputs=3
  MinMax2 : MinMax  Inputs=2
  ROOut2 : RelationalOperator  Operator===  OutDataTypeStr=boolean  RndMeth=Simplest
  Out1 : Outport
  wires:
  Data Type Conversion1/1 -> MinMax2/1
  MinMax2/1 -> MinMax/2, Memory2/1
  Memory2/1 -> MinMax2/2
  ROOut2/1 -> Data Type Conversion1/1
  [out2] -> ROOut2/2
  In2/1 -> ROOut2/1
  MinMax/1 -> Out1/1
  Constant1/1 -> MinMax/1
  Constant3/1 -> MinMax/3

== system c00017M_harness/Eval135 ==
  In2 : Inport
  Constant1 : Constant
  Constant3 : Constant
  Data Type Conversion1 : DataTypeConversion
  Memory2 : Memory  InitialCondition=1
  MinMax : MinMax  Inputs=3
  MinMax2 : MinMax  Inputs=2
  ROOut2 : RelationalOperator  Operator===  OutDataTypeStr=boolean  RndMeth=Simplest
  Out1 : Outport
  wires:
  Data Type Conversion1/1 -> MinMax2/1
  MinMax2/1 -> MinMax/2, Memory2/1
  Memory2/1 -> MinMax2/2
  ROOut2/1 -> Data Type Conversion1/1
  [out2] -> ROOut2/2
  In2/1 -> ROOut2/1
  MinMax/1 -> Out1/1
  Constant1/1 -> MinMax/1
  Constant3/1 -> MinMax/3

== system c00017M_harness/Eval136 ==
  In2 : Inport
  Constant1 : Constant
  Constant3 : Constant
  Data Type Conversion1 : DataTypeConversion
  Memory2 : Memory  InitialCondition=1
  MinMax : MinMax  Inputs=3
  MinMax2 : MinMax  Inputs=2
  ROOut2 : RelationalOperator  Operator===  OutDataTypeStr=boolean  RndMeth=Simplest
  Out1 : Outport
  wires:
  Data Type Conversion1/1 -> MinMax2/1
  MinMax2/1 -> MinMax/2, Memory2/1
  Memory2/1 -> MinMax2/2
  ROOut2/1 -> Data Type Conversion1/1
  [out2] -> ROOut2/2
  In2/1 -> ROOut2/1
  MinMax/1 -> Out1/1
  Constant1/1 -> MinMax/1
  Constant3/1 -> MinMax/3

== system c00017M_harness/Eval137 ==
  In2 : Inport
  Constant1 : Constant
  Constant3 : Constant
  Data Type Conversion1 : DataTypeConversion
  Memory2 : Memory  InitialCondition=1
  MinMax : MinMax  Inputs=3
  MinMax2 : MinMax  Inputs=2
  ROOut2 : RelationalOperator  Operator===  OutDataTypeStr=boolean  RndMeth=Simplest
  Out1 : Outport
  wires:
  Data Type Conversion1/1 -> MinMax2/1
  MinMax2/1 -> MinMax/2, Memory2/1
  Memory2/1 -> MinMax2/2
  ROOut2/1 -> Data Type Conversion1/1
  [out2] -> ROOut2/2
  In2/1 -> ROOut2/1
  MinMax/1 -> Out1/1
  Constant1/1 -> MinMax/1
  Constant3/1 -> MinMax/3

== system c00017M_harness/Eval139 ==
  In2 : Inport
  Constant1 : Constant
  Constant3 : Constant
  Data Type Conversion1 : DataTypeConversion
  Memory2 : Memory  InitialCondition=1
  MinMax : MinMax  Inputs=3
  MinMax2 : MinMax  Inputs=2
  ROOut2 : RelationalOperator  Operator===  OutDataTypeStr=boolean  RndMeth=Simplest
  Out1 : Outport
  wires:
  Data Type Conversion1/1 -> MinMax2/1
  MinMax2/1 -> MinMax/2, Memory2/1
  Memory2/1 -> MinMax2/2
  ROOut2/1 -> Data Type Conversion1/1
  [out2] -> ROOut2/2
  In2/1 -> ROOut2/1
  MinMax/1 -> Out1/1
  Constant1/1 -> MinMax/1
  Constant3/1 -> MinMax/3

== system c00017M_harness/Eval140 ==
  In2 : Inport
  Constant1 : Constant
  Constant3 : Constant
  Data Type Conversion1 : DataTypeConversion
  Memory2 : Memory  InitialCondition=1
  MinMax : MinMax  Inputs=3
  MinMax2 : MinMax  Inputs=2
  ROOut2 : RelationalOperator  Operator===  OutDataTypeStr=boolean  RndMeth=Simplest
  Out1 : Outport
  wires:
  Data Type Conversion1/1 -> MinMax2/1
  MinMax2/1 -> MinMax/2, Memory2/1
  Memory2/1 -> MinMax2/2
  ROOut2/1 -> Data Type Conversion1/1
  [out2] -> ROOut2/2
  In2/1 -> ROOut2/1
  MinMax/1 -> Out1/1
  Constant1/1 -> MinMax/1
  Constant3/1 -> MinMax/3

== system c00017M_harness/Eval141 ==
  In2 : Inport
  Constant1 : Constant
  Constant3 : Constant
  Data Type Conversion1 : DataTypeConversion
  Memory2 : Memory  InitialCondition=1
  MinMax : MinMax  Inputs=3
  MinMax2 : MinMax  Inputs=2
  ROOut2 : RelationalOperator  Operator===  OutDataTypeStr=boolean  RndMeth=Simplest
  Out1 : Outport
  wires:
  Data Type Conversion1/1 -> MinMax2/1
  MinMax2/1 -> MinMax/2, Memory2/1
  Memory2/1 -> MinMax2/2
  ROOut2/1 -> Data Type Conversion1/1
  [out2] -> ROOut2/2
  In2/1 -> ROOut2/1
  MinMax/1 -> Out1/1
  Constant1/1 -> MinMax/1
  Constant3/1 -> MinMax/3

== system c00017M_harness/Eval142 ==
  In2 : Inport
  Constant1 : Constant
  Constant3 : Constant
  Data Type Conversion1 : DataTypeConversion
  Memory2 : Memory  InitialCondition=1
  MinMax : MinMax  Inputs=3
  MinMax2 : MinMax  Inputs=2
  ROOut2 : RelationalOperator  Operator===  OutDataTypeStr=boolean  RndMeth=Simplest
  Out1 : Outport
  wires:
  Data Type Conversion1/1 -> MinMax2/1
  MinMax2/1 -> MinMax/2, Memory2/1
  Memory2/1 -> MinMax2/2
  ROOut2/1 -> Data Type Conversion1/1
  [out2] -> ROOut2/2
  In2/1 -> ROOut2/1
  MinMax/1 -> Out1/1
  Constant1/1 -> MinMax/1
  Constant3/1 -> MinMax/3

== system c00017M_harness/Eval150 ==
  In2 : Inport
  Constant1 : Constant
  Constant3 : Constant
  Data Type Conversion1 : DataTypeConversion
  Memory2 : Memory  InitialCondition=1
  MinMax : MinMax  Inputs=3
  MinMax2 : MinMax  Inputs=2
  ROOut2 : RelationalOperator  Operator===  OutDataTypeStr=boolean  RndMeth=Simplest
  Out1 : Outport
  wires:
  Data Type Conversion1/1 -> MinMax2/1
  MinMax2/1 -> MinMax/2, Memory2/1
  Memory2/1 -> MinMax2/2
  ROOut2/1 -> Data Type Conversion1/1
  [out2] -> ROOut2/2
  In2/1 -> ROOut2/1
  MinMax/1 -> Out1/1
  Constant1/1 -> MinMax/1
  Constant3/1 -> MinMax/3

== system c00017M_harness/Eval151 ==
  In2 : Inport
  Constant1 : Constant
  Constant3 : Constant
  Data Type Conversion1 : DataTypeConversion
  Memory2 : Memory  InitialCondition=1
  MinMax : MinMax  Inputs=3
  MinMax2 : MinMax  Inputs=2
  ROOut2 : RelationalOperator  Operator===  OutDataTypeStr=boolean  RndMeth=Simplest
  Out1 : Outport
  wires:
  Data Type Conversion1/1 -> MinMax2/1
  MinMax2/1 -> MinMax/2, Memory2/1
  Memory2/1 -> MinMax2/2
  ROOut2/1 -> Data Type Conversion1/1
  [out2] -> ROOut2/2
  In2/1 -> ROOut2/1
  MinMax/1 -> Out1/1
  Constant1/1 -> MinMax/1
  Constant3/1 -> MinMax/3

== system c00017M_harness/Eval152 ==
  In2 : Inport
  Constant1 : Constant
  Constant3 : Constant
  Data Type Conversion1 : DataTypeConversion
  Memory2 : Memory  InitialCondition=1
  MinMax : MinMax  Inputs=3
  MinMax2 : MinMax  Inputs=2
  ROOut2 : RelationalOperator  Operator===  OutDataTypeStr=boolean  RndMeth=Simplest
  Out1 : Outport
  wires:
  Data Type Conversion1/1 -> MinMax2/1
  MinMax2/1 -> MinMax/2, Memory2/1
  Memory2/1 -> MinMax2/2
  ROOut2/1 -> Data Type Conversion1/1
  [out2] -> ROOut2/2
  In2/1 -> ROOut2/1
  MinMax/1 -> Out1/1
  Constant1/1 -> MinMax/1
  Constant3/1 -> MinMax/3

== system c00017M_harness/Eval153 ==
  In2 : Inport
  Constant1 : Constant
  Constant3 : Constant
  Data Type Conversion1 : DataTypeConversion
  Memory2 : Memory  InitialCondition=1
  MinMax : MinMax  Inputs=3
  MinMax2 : MinMax  Inputs=2
  ROOut2 : RelationalOperator  Operator===  OutDataTypeStr=boolean  RndMeth=Simplest
  Out1 : Outport
  wires:
  Data Type Conversion1/1 -> MinMax2/1
  MinMax2/1 -> MinMax/2, Memory2/1
  Memory2/1 -> MinMax2/2
  ROOut2/1 -> Data Type Conversion1/1
  [out2] -> ROOut2/2
  In2/1 -> ROOut2/1
  MinMax/1 -> Out1/1
  Constant1/1 -> MinMax/1
  Constant3/1 -> MinMax/3

== system c00017M_harness/Eval154 ==
  In2 : Inport
  Constant1 : Constant
  Constant3 : Constant
  Data Type Conversion1 : DataTypeConversion
  Memory2 : Memory  InitialCondition=1
  MinMax : MinMax  Inputs=3
  MinMax2 : MinMax  Inputs=2
  ROOut2 : RelationalOperator  Operator===  OutDataTypeStr=boolean  RndMeth=Simplest
  Out1 : Outport
  wires:
  Data Type Conversion1/1 -> MinMax2/1
  MinMax2/1 -> MinMax/2, Memory2/1
  Memory2/1 -> MinMax2/2
  ROOut2/1 -> Data Type Conversion1/1
  [out2] -> ROOut2/2
  In2/1 -> ROOut2/1
  MinMax/1 -> Out1/1
  Constant1/1 -> MinMax/1
  Constant3/1 -> MinMax/3

== system c00017M_harness/Eval155 ==
  In2 : Inport
  Constant1 : Constant
  Constant3 : Constant
  Data Type Conversion1 : DataTypeConversion
  Memory2 : Memory  InitialCondition=1
  MinMax : MinMax  Inputs=3
  MinMax2 : MinMax  Inputs=2
  ROOut2 : RelationalOperator  Operator===  OutDataTypeStr=boolean  RndMeth=Simplest
  Out1 : Outport
  wires:
  Data Type Conversion1/1 -> MinMax2/1
  MinMax2/1 -> MinMax/2, Memory2/1
  Memory2/1 -> MinMax2/2
  ROOut2/1 -> Data Type Conversion1/1
  [out2] -> ROOut2/2
  In2/1 -> ROOut2/1
  MinMax/1 -> Out1/1
  Constant1/1 -> MinMax/1
  Constant3/1 -> MinMax/3

== system c00017M_harness/Eval156 ==
  In2 : Inport
  Constant1 : Constant
  Constant3 : Constant
  Data Type Conversion1 : DataTypeConversion
  Memory2 : Memory  InitialCondition=1
  MinMax : MinMax  Inputs=3
  MinMax2 : MinMax  Inputs=2
  ROOut2 : RelationalOperator  Operator===  OutDataTypeStr=boolean  RndMeth=Simplest
  Out1 : Outport
  wires:
  Data Type Conversion1/1 -> MinMax2/1
  MinMax2/1 -> MinMax/2, Memory2/1
  Memory2/1 -> MinMax2/2
  ROOut2/1 -> Data Type Conversion1/1
  [out2] -> ROOut2/2
  In2/1 -> ROOut2/1
  MinMax/1 -> Out1/1
  Constant1/1 -> MinMax/1
  Constant3/1 -> MinMax/3

== system c00017M_harness/Eval157 ==
  In2 : Inport
  Constant1 : Constant
  Constant3 : Constant
  Data Type Conversion1 : DataTypeConversion
  Memory2 : Memory  InitialCondition=1
  MinMax : MinMax  Inputs=3
  MinMax2 : MinMax  Inputs=2
  ROOut2 : RelationalOperator  Operator===  OutDataTypeStr=boolean  RndMeth=Simplest
  Out1 : Outport
  wires:
  Data Type Conversion1/1 -> MinMax2/1
  MinMax2/1 -> MinMax/2, Memory2/1
  Memory2/1 -> MinMax2/2
  ROOut2/1 -> Data Type Conversion1/1
  [out2] -> ROOut2/2
  In2/1 -> ROOut2/1
  MinMax/1 -> Out1/1
  Constant1/1 -> MinMax/1
  Constant3/1 -> MinMax/3

== system c00017M_harness/Eval158 ==
  In2 : Inport
  Constant1 : Constant
  Constant3 : Constant
  Data Type Conversion1 : DataTypeConversion
  Memory2 : Memory  InitialCondition=1
  MinMax : MinMax  Inputs=3
  MinMax2 : MinMax  Inputs=2
  ROOut2 : RelationalOperator  Operator===  OutDataTypeStr=boolean  RndMeth=Simplest
  Out1 : Outport
  wires:
  Data Type Conversion1/1 -> MinMax2/1
  MinMax2/1 -> MinMax/2, Memory2/1
  Memory2/1 -> MinMax2/2
  ROOut2/1 -> Data Type Conversion1/1
  [out2] -> ROOut2/2
  In2/1 -> ROOut2/1
  MinMax/1 -> Out1/1
  Constant1/1 -> MinMax/1
  Constant3/1 -> MinMax/3

== system c00017M_harness/Eval159 ==
  In2 : Inport
  Constant1 : Constant
  Constant3 : Constant
  Data Type Conversion1 : DataTypeConversion
  Memory2 : Memory  InitialCondition=1
  MinMax : MinMax  Inputs=3
  MinMax2 : MinMax  Inputs=2
  ROOut2 : RelationalOperator  Operator===  OutDataTypeStr=boolean  RndMeth=Simplest
  Out1 : Outport
  wires:
  Data Type Conversion1/1 -> MinMax2/1
  MinMax2/1 -> MinMax/2, Memory2/1
  Memory2/1 -> MinMax2/2
  ROOut2/1 -> Data Type Conversion1/1
  [out2] -> ROOut2/2
  In2/1 -> ROOut2/1
  MinMax/1 -> Out1/1
  Constant1/1 -> MinMax/1
  Constant3/1 -> MinMax/3

== system c00017M_harness/Eval160 ==
  In2 : Inport
  Constant1 : Constant
  Constant3 : Constant
  Data Type Conversion1 : DataTypeConversion
  Memory2 : Memory  InitialCondition=1
  MinMax : MinMax  Inputs=3
  MinMax2 : MinMax  Inputs=2
  ROOut2 : RelationalOperator  Operator===  OutDataTypeStr=boolean  RndMeth=Simplest
  Out1 : Outport
  wires:
  Data Type Conversion1/1 -> MinMax2/1
  MinMax2/1 -> MinMax/2, Memory2/1
  Memory2/1 -> MinMax2/2
  ROOut2/1 -> Data Type Conversion1/1
  [out2] -> ROOut2/2
  In2/1 -> ROOut2/1
  MinMax/1 -> Out1/1
  Constant1/1 -> MinMax/1
  Constant3/1 -> MinMax/3

== system c00017M_harness/Eval161 ==
  In2 : Inport
  Constant1 : Constant
  Constant3 : Constant
  Data Type Conversion1 : DataTypeConversion
  Memory2 : Memory  InitialCondition=1
  MinMax : MinMax  Inputs=3
  MinMax2 : MinMax  Inputs=2
  ROOut2 : RelationalOperator  Operator===  OutDataTypeStr=boolean  RndMeth=Simplest
  Out1 : Outport
  wires:
  Data Type Conversion1/1 -> MinMax2/1
  MinMax2/1 -> MinMax/2, Memory2/1
  Memory2/1 -> MinMax2/2
  ROOut2/1 -> Data Type Conversion1/1
  [out2] -> ROOut2/2
  In2/1 -> ROOut2/1
  MinMax/1 -> Out1/1
  Constant1/1 -> MinMax/1
  Constant3/1 -> MinMax/3

== system c00017M_harness/Eval162 ==
  In2 : Inport
  Constant1 : Constant
  Constant3 : Constant
  Data Type Conversion1 : DataTypeConversion
  Memory2 : Memory  InitialCondition=1
  MinMax : MinMax  Inputs=3
  MinMax2 : MinMax  Inputs=2
  ROOut2 : RelationalOperator  Operator===  OutDataTypeStr=boolean  RndMeth=Simplest
  Out1 : Outport
  wires:
  Data Type Conversion1/1 -> MinMax2/1
  MinMax2/1 -> MinMax/2, Memory2/1
  Memory2/1 -> MinMax2/2
  ROOut2/1 -> Data Type Conversion1/1
  [out2] -> ROOut2/2
  In2/1 -> ROOut2/1
  MinMax/1 -> Out1/1
  Constant1/1 -> MinMax/1
  Constant3/1 -> MinMax/3

== system c00017M_harness/Eval163 ==
  In2 : Inport
  Constant1 : Constant
  Constant3 : Constant
  Data Type Conversion1 : DataTypeConversion
  Memory2 : Memory  InitialCondition=1
  MinMax : MinMax  Inputs=3
  MinMax2 : MinMax  Inputs=2
  ROOut2 : RelationalOperator  Operator===  OutDataTypeStr=boolean  RndMeth=Simplest
  Out1 : Outport
  wires:
  Data Type Conversion1/1 -> MinMax2/1
  MinMax2/1 -> MinMax/2, Memory2/1
  Memory2/1 -> MinMax2/2
  ROOut2/1 -> Data Type Conversion1/1
  [out2] -> ROOut2/2
  In2/1 -> ROOut2/1
  MinMax/1 -> Out1/1
  Constant1/1 -> MinMax/1
  Constant3/1 -> MinMax/3

== system c00017M_harness/Eval82 ==
  In2 : Inport
  Constant1 : Constant
  Constant3 : Constant
  Data Type Conversion1 : DataTypeConversion
  Memory2 : Memory  InitialCondition=1
  MinMax : MinMax  Inputs=3
  MinMax2 : MinMax  Inputs=2
  ROOut2 : RelationalOperator  Operator===  OutDataTypeStr=boolean  RndMeth=Simplest
  Out1 : Outport
  wires:
  Data Type Conversion1/1 -> MinMax2/1
  MinMax2/1 -> MinMax/2, Memory2/1
  Memory2/1 -> MinMax2/2
  ROOut2/1 -> Data Type Conversion1/1
  [out2] -> ROOut2/2
  In2/1 -> ROOut2/1
  MinMax/1 -> Out1/1
  Constant1/1 -> MinMax/1
  Constant3/1 -> MinMax/3

== system c00017M_harness/Inputs ==
  Demux : Demux  Tag=STV Demux  Outputs=6
  FromWs : FromWorkspace  Tag=STV FromWs  VariableName=tuvar  SampleTime=0
  CT2 : Outport  Tag=STV Outport
  F2 : Outport  Tag=STV Outport  Port=2
  E2 : Outport  Tag=STV Outport  Port=3
  MR2 : Outport  Tag=STV Outport  Port=4
  T2 : Outport  Tag=STV Outport  Port=5
  EB2 : Outport  Tag=STV Outport  Port=6
  wires:
  Demux/6 -> EB2/1
  Demux/5 -> T2/1
  Demux/4 -> MR2/1
  Demux/3 -> E2/1
  Demux/2 -> F2/1
  Demux/1 -> CT2/1
  FromWs/1 -> Demux/1

== system c00017M_harness/M083 ==
  note: VALUES
      | ---------------------------------
      | ControlType = 1 | 2 | 3
      | FillTank = 0 | 1
      | EmptyTank = 0 | 1
      | ManualReference between 0 and 1
      | Tempreature between 0 and 100
      | EmergencyButton = 0 | 1
      | LiquidLevel between 0 and 1 (hmax)
  note: Inputs For Tank2
  note: NAMES
      | --------------------------------------------
      | CT1 = ControlType Tank 1
      | F1 = Fill Tank 1
      | E1 = Empty Tank 1
      | MR1 = Manual Reference Tank1
      | T1 = Temperature Tank 1
      | EB1 = Emergency Button Tank 1
      | LL1 = Liquid Level 1
  note: Inputs For Tank3
  note: Inputs For Tank1
  CT2 : Inport
  F2 : Inport  Port=2
  E2 : Inport  Port=3
  MR2 : Inport  Port=4
  T2 : Inport  Port=5
  EB2 : Inport  Port=6
  Tank2 : Subsystem
  LL2 : Outport
  wires:
  Tank2/1(LL2) -> LL2/1
  EB2/1 -> Tank2/6(EB2)
  CT2/1 -> Tank2/1(CT2)
  F2/1 -> Tank2/2(F2)
  E2/1 -> Tank2/3(E2)
  T2/1 -> Tank2/5(T2)
  MR2/1 -> Tank2/4(MR2)

== system c00017M_harness/M118 ==
  note: VALUES
      | ---------------------------------
      | ControlType = 1 | 2 | 3
      | FillTank = 0 | 1
      | EmptyTank = 0 | 1
      | ManualReference between 0 and 1
      | Tempreature between 0 and 100
      | EmergencyButton = 0 | 1
      | LiquidLevel between 0 and 1 (hmax)
  note: Inputs For Tank2
  note: NAMES
      | --------------------------------------------
      | CT1 = ControlType Tank 1
      | F1 = Fill Tank 1
      | E1 = Empty Tank 1
      | MR1 = Manual Reference Tank1
      | T1 = Temperature Tank 1
      | EB1 = Emergency Button Tank 1
      | LL1 = Liquid Level 1
  note: Inputs For Tank3
  note: Inputs For Tank1
  CT2 : Inport
  F2 : Inport  Port=2
  E2 : Inport  Port=3
  MR2 : Inport  Port=4
  T2 : Inport  Port=5
  EB2 : Inport  Port=6
  Tank2 : Subsystem
  LL2 : Outport
  wires:
  Tank2/1(LL2) -> LL2/1
  EB2/1 -> Tank2/6(EB2)
  CT2/1 -> Tank2/1(CT2)
  F2/1 -> Tank2/2(F2)
  E2/1 -> Tank2/3(E2)
  T2/1 -> Tank2/5(T2)
  MR2/1 -> Tank2/4(MR2)

== system c00017M_harness/M119 ==
  note: VALUES
      | ---------------------------------
      | ControlType = 1 | 2 | 3
      | FillTank = 0 | 1
      | EmptyTank = 0 | 1
      | ManualReference between 0 and 1
      | Tempreature between 0 and 100
      | EmergencyButton = 0 | 1
      | LiquidLevel between 0 and 1 (hmax)
  note: Inputs For Tank2
  note: NAMES
      | --------------------------------------------
      | CT1 = ControlType Tank 1
      | F1 = Fill Tank 1
      | E1 = Empty Tank 1
      | MR1 = Manual Reference Tank1
      | T1 = Temperature Tank 1
      | EB1 = Emergency Button Tank 1
      | LL1 = Liquid Level 1
  note: Inputs For Tank3
  note: Inputs For Tank1
  CT2 : Inport
  F2 : Inport  Port=2
  E2 : Inport  Port=3
  MR2 : Inport  Port=4
  T2 : Inport  Port=5
  EB2 : Inport  Port=6
  Tank2 : Subsystem
  LL2 : Outport
  wires:
  Tank2/1(LL2) -> LL2/1
  EB2/1 -> Tank2/6(EB2)
  CT2/1 -> Tank2/1(CT2)
  F2/1 -> Tank2/2(F2)
  E2/1 -> Tank2/3(E2)
  T2/1 -> Tank2/5(T2)
  MR2/1 -> Tank2/4(MR2)

== system c00017M_harness/M120 ==
  note: VALUES
      | ---------------------------------
      | ControlType = 1 | 2 | 3
      | FillTank = 0 | 1
      | EmptyTank = 0 | 1
      | ManualReference between 0 and 1
      | Tempreature between 0 and 100
      | EmergencyButton = 0 | 1
      | LiquidLevel between 0 and 1 (hmax)
  note: Inputs For Tank2
  note: NAMES
      | --------------------------------------------
      | CT1 = ControlType Tank 1
      | F1 = Fill Tank 1
      | E1 = Empty Tank 1
      | MR1 = Manual Reference Tank1
      | T1 = Temperature Tank 1
      | EB1 = Emergency Button Tank 1
      | LL1 = Liquid Level 1
  note: Inputs For Tank3
  note: Inputs For Tank1
  CT2 : Inport
  F2 : Inport  Port=2
  E2 : Inport  Port=3
  MR2 : Inport  Port=4
  T2 : Inport  Port=5
  EB2 : Inport  Port=6
  Tank2 : Subsystem
  LL2 : Outport
  wires:
  Tank2/1(LL2) -> LL2/1
  EB2/1 -> Tank2/6(EB2)
  CT2/1 -> Tank2/1(CT2)
  F2/1 -> Tank2/2(F2)
  E2/1 -> Tank2/3(E2)
  T2/1 -> Tank2/5(T2)
  MR2/1 -> Tank2/4(MR2)

== system c00017M_harness/M121 ==
  note: VALUES
      | ---------------------------------
      | ControlType = 1 | 2 | 3
      | FillTank = 0 | 1
      | EmptyTank = 0 | 1
      | ManualReference between 0 and 1
      | Tempreature between 0 and 100
      | EmergencyButton = 0 | 1
      | LiquidLevel between 0 and 1 (hmax)
  note: Inputs For Tank2
  note: NAMES
      | --------------------------------------------
      | CT1 = ControlType Tank 1
      | F1 = Fill Tank 1
      | E1 = Empty Tank 1
      | MR1 = Manual Reference Tank1
      | T1 = Temperature Tank 1
      | EB1 = Emergency Button Tank 1
      | LL1 = Liquid Level 1
  note: Inputs For Tank3
  note: Inputs For Tank1
  CT2 : Inport
  F2 : Inport  Port=2
  E2 : Inport  Port=3
  MR2 : Inport  Port=4
  T2 : Inport  Port=5
  EB2 : Inport  Port=6
  Tank2 : Subsystem
  LL2 : Outport
  wires:
  Tank2/1(LL2) -> LL2/1
  EB2/1 -> Tank2/6(EB2)
  CT2/1 -> Tank2/1(CT2)
  F2/1 -> Tank2/2(F2)
  E2/1 -> Tank2/3(E2)
  T2/1 -> Tank2/5(T2)
  MR2/1 -> Tank2/4(MR2)

== system c00017M_harness/M122 ==
  note: VALUES
      | ---------------------------------
      | ControlType = 1 | 2 | 3
      | FillTank = 0 | 1
      | EmptyTank = 0 | 1
      | ManualReference between 0 and 1
      | Tempreature between 0 and 100
      | EmergencyButton = 0 | 1
      | LiquidLevel between 0 and 1 (hmax)
  note: Inputs For Tank2
  note: NAMES
      | --------------------------------------------
      | CT1 = ControlType Tank 1
      | F1 = Fill Tank 1
      | E1 = Empty Tank 1
      | MR1 = Manual Reference Tank1
      | T1 = Temperature Tank 1
      | EB1 = Emergency Button Tank 1
      | LL1 = Liquid Level 1
  note: Inputs For Tank3
  note: Inputs For Tank1
  CT2 : Inport
  F2 : Inport  Port=2
  E2 : Inport  Port=3
  MR2 : Inport  Port=4
  T2 : Inport  Port=5
  EB2 : Inport  Port=6
  Tank2 : Subsystem
  LL2 : Outport
  wires:
  Tank2/1(LL2) -> LL2/1
  EB2/1 -> Tank2/6(EB2)
  CT2/1 -> Tank2/1(CT2)
  F2/1 -> Tank2/2(F2)
  E2/1 -> Tank2/3(E2)
  T2/1 -> Tank2/5(T2)
  MR2/1 -> Tank2/4(MR2)

== system c00017M_harness/M123 ==
  note: VALUES
      | ---------------------------------
      | ControlType = 1 | 2 | 3
      | FillTank = 0 | 1
      | EmptyTank = 0 | 1
      | ManualReference between 0 and 1
      | Tempreature between 0 and 100
      | EmergencyButton = 0 | 1
      | LiquidLevel between 0 and 1 (hmax)
  note: Inputs For Tank2
  note: NAMES
      | --------------------------------------------
      | CT1 = ControlType Tank 1
      | F1 = Fill Tank 1
      | E1 = Empty Tank 1
      | MR1 = Manual Reference Tank1
      | T1 = Temperature Tank 1
      | EB1 = Emergency Button Tank 1
      | LL1 = Liquid Level 1
  note: Inputs For Tank3
  note: Inputs For Tank1
  CT2 : Inport
  F2 : Inport  Port=2
  E2 : Inport  Port=3
  MR2 : Inport  Port=4
  T2 : Inport  Port=5
  EB2 : Inport  Port=6
  Tank2 : Subsystem
  LL2 : Outport
  wires:
  Tank2/1(LL2) -> LL2/1
  EB2/1 -> Tank2/6(EB2)
  CT2/1 -> Tank2/1(CT2)
  F2/1 -> Tank2/2(F2)
  E2/1 -> Tank2/3(E2)
  T2/1 -> Tank2/5(T2)
  MR2/1 -> Tank2/4(MR2)

== system c00017M_harness/M124 ==
  note: VALUES
      | ---------------------------------
      | ControlType = 1 | 2 | 3
      | FillTank = 0 | 1
      | EmptyTank = 0 | 1
      | ManualReference between 0 and 1
      | Tempreature between 0 and 100
      | EmergencyButton = 0 | 1
      | LiquidLevel between 0 and 1 (hmax)
  note: Inputs For Tank2
  note: NAMES
      | --------------------------------------------
      | CT1 = ControlType Tank 1
      | F1 = Fill Tank 1
      | E1 = Empty Tank 1
      | MR1 = Manual Reference Tank1
      | T1 = Temperature Tank 1
      | EB1 = Emergency Button Tank 1
      | LL1 = Liquid Level 1
  note: Inputs For Tank3
  note: Inputs For Tank1
  CT2 : Inport
  F2 : Inport  Port=2
  E2 : Inport  Port=3
  MR2 : Inport  Port=4
  T2 : Inport  Port=5
  EB2 : Inport  Port=6
  Tank2 : Subsystem
  LL2 : Outport
  wires:
  Tank2/1(LL2) -> LL2/1
  EB2/1 -> Tank2/6(EB2)
  CT2/1 -> Tank2/1(CT2)
  F2/1 -> Tank2/2(F2)
  E2/1 -> Tank2/3(E2)
  T2/1 -> Tank2/5(T2)
  MR2/1 -> Tank2/4(MR2)

== system c00017M_harness/M125 ==
  note: VALUES
      | ---------------------------------
      | ControlType = 1 | 2 | 3
      | FillTank = 0 | 1
      | EmptyTank = 0 | 1
      | ManualReference between 0 and 1
      | Tempreature between 0 and 100
      | EmergencyButton = 0 | 1
      | LiquidLevel between 0 and 1 (hmax)
  note: Inputs For Tank2
  note: NAMES
      | --------------------------------------------
      | CT1 = ControlType Tank 1
      | F1 = Fill Tank 1
      | E1 = Empty Tank 1
      | MR1 = Manual Reference Tank1
      | T1 = Temperature Tank 1
      | EB1 = Emergency Button Tank 1
      | LL1 = Liquid Level 1
  note: Inputs For Tank3
  note: Inputs For Tank1
  CT2 : Inport
  F2 : Inport  Port=2
  E2 : Inport  Port=3
  MR2 : Inport  Port=4
  T2 : Inport  Port=5
  EB2 : Inport  Port=6
  Tank2 : Subsystem
  LL2 : Outport
  wires:
  Tank2/1(LL2) -> LL2/1
  EB2/1 -> Tank2/6(EB2)
  CT2/1 -> Tank2/1(CT2)
  F2/1 -> Tank2/2(F2)
  E2/1 -> Tank2/3(E2)
  T2/1 -> Tank2/5(T2)
  MR2/1 -> Tank2/4(MR2)

== system c00017M_harness/M126 ==
  note: VALUES
      | ---------------------------------
      | ControlType = 1 | 2 | 3
      | FillTank = 0 | 1
      | EmptyTank = 0 | 1
      | ManualReference between 0 and 1
      | Tempreature between 0 and 100
      | EmergencyButton = 0 | 1
      | LiquidLevel between 0 and 1 (hmax)
  note: Inputs For Tank2
  note: NAMES
      | --------------------------------------------
      | CT1 = ControlType Tank 1
      | F1 = Fill Tank 1
      | E1 = Empty Tank 1
      | MR1 = Manual Reference Tank1
      | T1 = Temperature Tank 1
      | EB1 = Emergency Button Tank 1
      | LL1 = Liquid Level 1
  note: Inputs For Tank3
  note: Inputs For Tank1
  CT2 : Inport
  F2 : Inport  Port=2
  E2 : Inport  Port=3
  MR2 : Inport  Port=4
  T2 : Inport  Port=5
  EB2 : Inport  Port=6
  Tank2 : Subsystem
  LL2 : Outport
  wires:
  Tank2/1(LL2) -> LL2/1
  EB2/1 -> Tank2/6(EB2)
  CT2/1 -> Tank2/1(CT2)
  F2/1 -> Tank2/2(F2)
  E2/1 -> Tank2/3(E2)
  T2/1 -> Tank2/5(T2)
  MR2/1 -> Tank2/4(MR2)
